simulink model "Lab3Kinematics"  (R2024a)
settings: Solver=VariableStepAuto  StartTime=0.0  StopTime=10.0  RelTol=1e-3
model workspace (MAT data in the model file):
  L = Simulink.Parameter
  L.Value = 0.1
  L.Complexity = 'real'
  L.Dimensions = [1 1]
  L.DataType = 'auto'
  r = Simulink.Parameter
  r.Value = 0.03
  r.Complexity = 'real'
  r.Dimensions = [1 1]
  r.DataType = 'auto'
settings Model: Creator=qjaus  LastModifiedBy=Beast

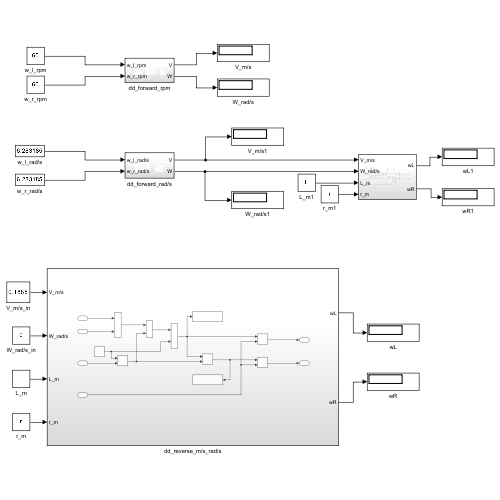
[thumbnail: Simulink's stored preview of the top-level diagram]
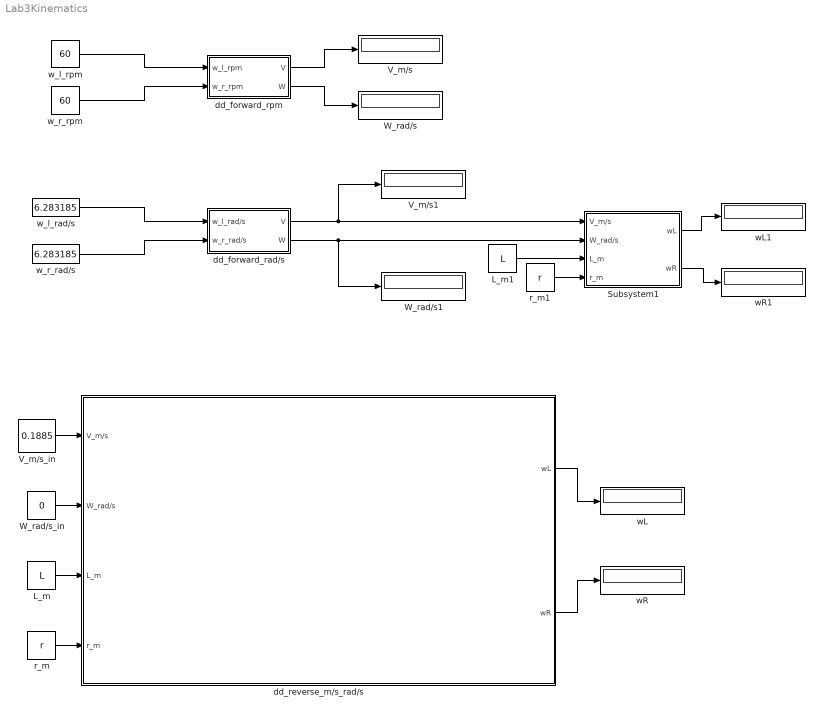
== system Lab3Kinematics ==
  L_m : Constant  Value=L
  L_m1 : Constant  Value=L
  Subsystem1 : Subsystem
  V_m/s : Display
  V_m/s1 : Display
  V_m/s_in : Constant  Value=0.1885
  W_rad/s : Display
  W_rad/s1 : Display
  W_rad/s_in : Constant  Value=0
  dd_forward_rad/s : Subsystem
  dd_forward_rpm : Subsystem
  dd_reverse_m/s_rad/s : Subsystem
  r_m : Constant  Value=r
  r_m1 : Constant  Value=r
  wL : Display
  wL1 : Display
  wR : Display
  wR1 : Display
  w_l_rad/s : Constant  Value=6.283185
  w_l_rpm : Constant  Value=60
  w_r_rad/s : Constant  Value=6.283185
  w_r_rpm : Constant  Value=60
  wires:
  w_l_rpm/1 -> dd_forward_rpm/1(w_l_rpm)
  w_r_rpm/1 -> dd_forward_rpm/2(w_r_rpm)
  dd_forward_rpm/1(V) -> V_m/s/1
  dd_forward_rpm/2(W) -> W_rad/s/1
  dd_forward_rad/s/2(W) -> W_rad/s1/1, Subsystem1/2(W_rad/s)
  w_r_rad/s/1 -> dd_forward_rad/s/2(w_r_rad/s)
  w_l_rad/s/1 -> dd_forward_rad/s/1(w_l_rad/s)
  W_rad/s_in/1 -> dd_reverse_m/s_rad/s/2(W_rad/s)
  L_m/1 -> dd_reverse_m/s_rad/s/3(L_m)
  r_m/1 -> dd_reverse_m/s_rad/s/4(r_m)
  dd_reverse_m/s_rad/s/1(wL) -> wL/1
  dd_reverse_m/s_rad/s/2(wR) -> wR/1
  r_m1/1 -> Subsystem1/4(r_m)
  L_m1/1 -> Subsystem1/3(L_m)
  Subsystem1/1(wL) -> wL1/1
  Subsystem1/2(wR) -> wR1/1
  V_m/s_in/1 -> dd_reverse_m/s_rad/s/1(V_m/s)
  dd_forward_rad/s/1(V) -> V_m/s1/1, Subsystem1/1(V_m/s)

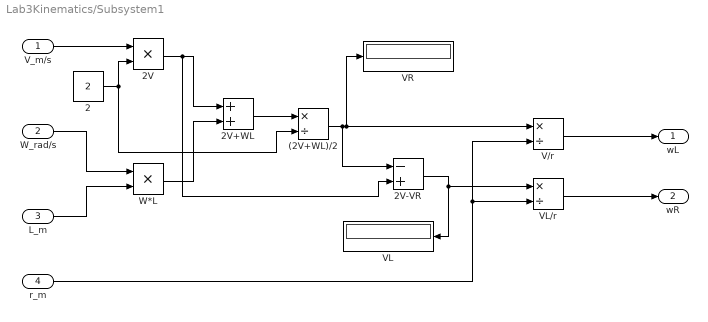
== system Lab3Kinematics/Subsystem1 ==
  V_m/s : Inport
  W_rad/s : Inport  Port=2
  L_m : Inport  Port=3
  r_m : Inport  Port=4
  (2V+WL)/2 : Product  Inputs=*/
  2 : Constant  Value=2
  2V : Product
  2V+WL : Sum
  2V-VR : Sum  Inputs=-+
  V/r : Product  Inputs=*/
  VL : Display
  VL/r : Product  Inputs=*/
  VR : Display
  W*L : Product
  wL : Outport
  wR : Outport  Port=2
  wires:
  2/1 -> 2V/2, (2V+WL)/2/2
  W*L/1 -> 2V+WL/2
  (2V+WL)/2/1 -> 2V-VR/1, VR/1, V/r/1
  r_m/1 -> V/r/2, VL/r/2
  2V-VR/1 -> VL/1, VL/r/1
  2V/1 -> 2V+WL/1, 2V-VR/2
  VL/r/1 -> wR/1
  2V+WL/1 -> (2V+WL)/2/1
  V/r/1 -> wL/1
  V_m/s/1 -> 2V/1
  W_rad/s/1 -> W*L/1
  L_m/1 -> W*L/2

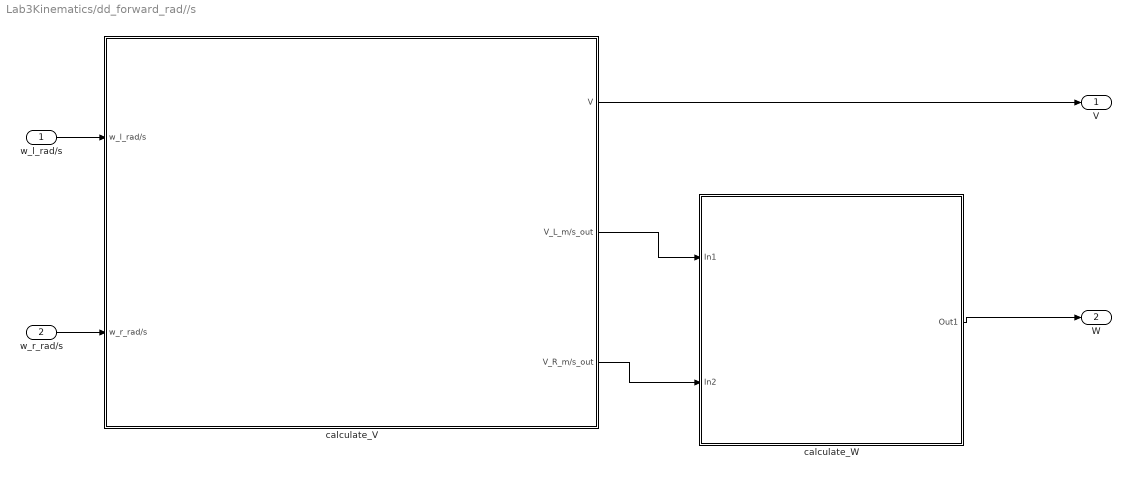
== system Lab3Kinematics/dd_forward_rad//s ==
  w_l_rad/s : Inport
  w_r_rad/s : Inport  Port=2
  calculate_V : Subsystem
  calculate_W : Subsystem
  V : Outport
  W : Outport  Port=2
  wires:
  calculate_V/1(V) -> V/1
  w_r_rad/s/1 -> calculate_V/2(w_r_rad/s)
  w_l_rad/s/1 -> calculate_V/1(w_l_rad/s)
  calculate_V/2(V_L_m/s_out) -> calculate_W/1(In1)
  calculate_W/1(Out1) -> W/1
  calculate_V/3(V_R_m/s_out) -> calculate_W/2(In2)

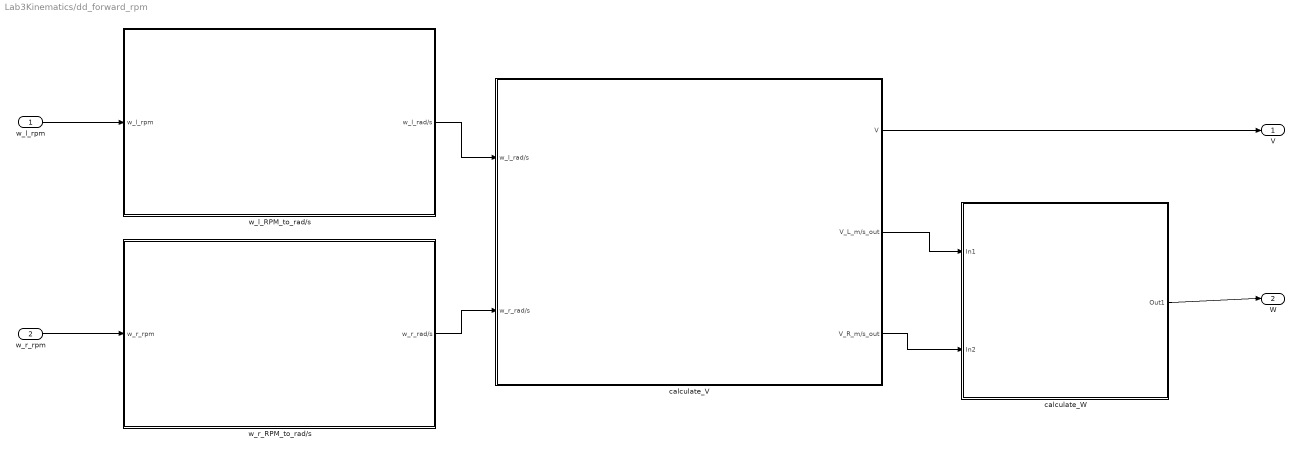
== system Lab3Kinematics/dd_forward_rpm ==
  w_l_rpm : Inport
  w_r_rpm : Inport  Port=2
  calculate_V : Subsystem
  calculate_W : Subsystem
  w_l_RPM_to_rad/s : Subsystem
  w_r_RPM_to_rad/s : Subsystem
  V : Outport
  W : Outport  Port=2
  wires:
  calculate_V/1(V) -> V/1
  w_r_RPM_to_rad/s/1(w_r_rad/s) -> calculate_V/2(w_r_rad/s)
  w_l_RPM_to_rad/s/1(w_l_rad/s) -> calculate_V/1(w_l_rad/s)
  calculate_V/2(V_L_m/s_out) -> calculate_W/1(In1)
  calculate_W/1(Out1) -> W/1
  calculate_V/3(V_R_m/s_out) -> calculate_W/2(In2)
  w_l_rpm/1 -> w_l_RPM_to_rad/s/1(w_l_rpm)
  w_r_rpm/1 -> w_r_RPM_to_rad/s/1(w_r_rpm)

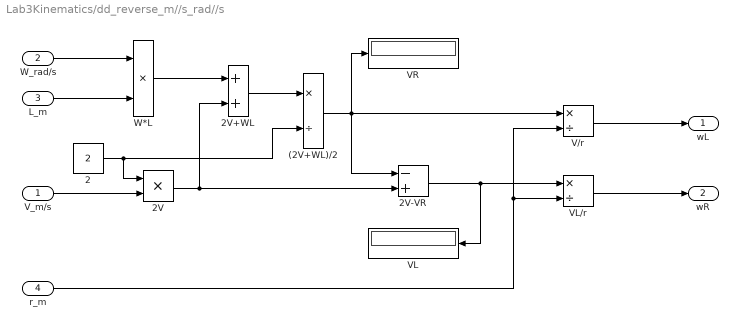
== system Lab3Kinematics/dd_reverse_m//s_rad//s ==
  V_m/s : Inport
  W_rad/s : Inport  Port=2
  L_m : Inport  Port=3
  r_m : Inport  Port=4
  (2V+WL)/2 : Product  Inputs=*/
  2 : Constant  Value=2
  2V : Product
  2V+WL : Sum
  2V-VR : Sum  Inputs=-+
  V/r : Product  Inputs=*/
  VL : Display
  VL/r : Product  Inputs=*/
  VR : Display
  W*L : Product
  wL : Outport
  wR : Outport  Port=2
  wires:
  2/1 -> 2V/1, (2V+WL)/2/2
  W*L/1 -> 2V+WL/1
  (2V+WL)/2/1 -> 2V-VR/1, V/r/1, VR/1
  r_m/1 -> V/r/2, VL/r/2
  2V-VR/1 -> VL/r/1, VL/1
  2V/1 -> 2V+WL/2, 2V-VR/2
  VL/r/1 -> wR/1
  2V+WL/1 -> (2V+WL)/2/1
  V/r/1 -> wL/1
  V_m/s/1 -> 2V/2
  W_rad/s/1 -> W*L/1
  L_m/1 -> W*L/2

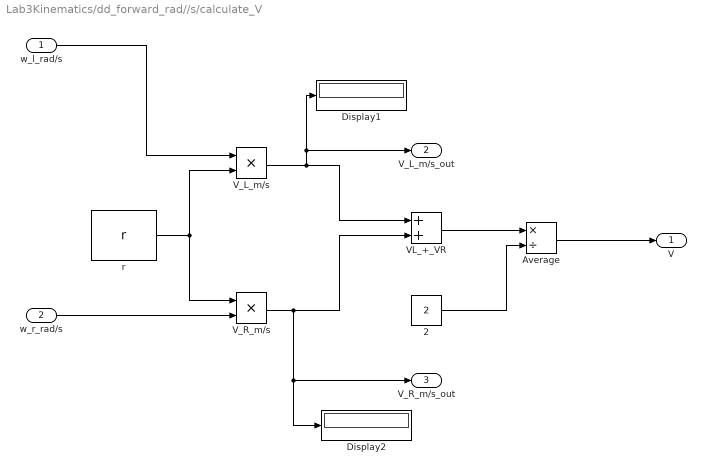
== system Lab3Kinematics/dd_forward_rad//s/calculate_V ==
  w_l_rad/s : Inport
  w_r_rad/s : Inport  Port=2
  2 : Constant  Value=2
  Average : Product  Inputs=*/
  Display1 : Display
  Display2 : Display
  VL_+_VR : Sum
  V_L_m/s : Product
  V_R_m/s : Product
  r : Constant  Value=r
  V : Outport
  V_L_m/s_out : Outport  Port=2
  V_R_m/s_out : Outport  Port=3
  wires:
  w_r_rad/s/1 -> V_R_m/s/2
  VL_+_VR/1 -> Average/1
  r/1 -> V_L_m/s/2, V_R_m/s/1
  V_L_m/s/1 -> Display1/1, V_L_m/s_out/1, VL_+_VR/1
  V_R_m/s/1 -> V_R_m/s_out/1, Display2/1, VL_+_VR/2
  2/1 -> Average/2
  w_l_rad/s/1 -> V_L_m/s/1
  Average/1 -> V/1

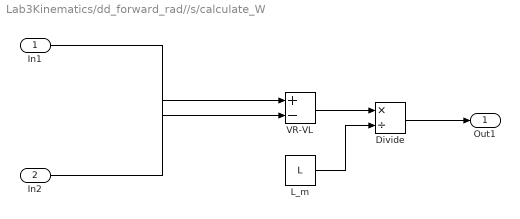
== system Lab3Kinematics/dd_forward_rad//s/calculate_W ==
  In1 : Inport
  In2 : Inport  Port=2
  Divide : Product  Inputs=*/
  L_m : Constant  Value=L
  VR-VL : Sum  Inputs=+-
  Out1 : Outport
  wires:
  L_m/1 -> Divide/2
  VR-VL/1 -> Divide/1
  In2/1 -> VR-VL/1
  In1/1 -> VR-VL/2
  Divide/1 -> Out1/1

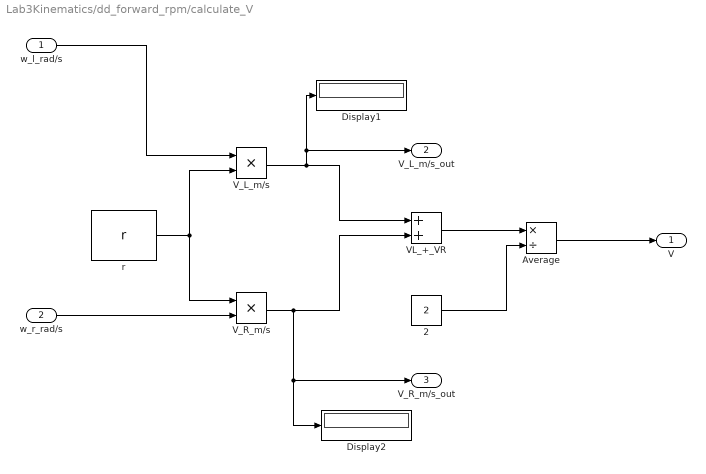
== system Lab3Kinematics/dd_forward_rpm/calculate_V ==
  w_l_rad/s : Inport
  w_r_rad/s : Inport  Port=2
  2 : Constant  Value=2
  Average : Product  Inputs=*/
  Display1 : Display
  Display2 : Display
  VL_+_VR : Sum
  V_L_m/s : Product
  V_R_m/s : Product
  r : Constant  Value=r
  V : Outport
  V_L_m/s_out : Outport  Port=2
  V_R_m/s_out : Outport  Port=3
  wires:
  w_r_rad/s/1 -> V_R_m/s/2
  VL_+_VR/1 -> Average/1
  r/1 -> V_L_m/s/2, V_R_m/s/1
  V_L_m/s/1 -> Display1/1, V_L_m/s_out/1, VL_+_VR/1
  V_R_m/s/1 -> V_R_m/s_out/1, Display2/1, VL_+_VR/2
  2/1 -> Average/2
  w_l_rad/s/1 -> V_L_m/s/1
  Average/1 -> V/1

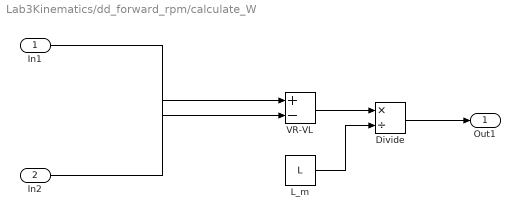
== system Lab3Kinematics/dd_forward_rpm/calculate_W ==
  In1 : Inport
  In2 : Inport  Port=2
  Divide : Product  Inputs=*/
  L_m : Constant  Value=L
  VR-VL : Sum  Inputs=+-
  Out1 : Outport
  wires:
  L_m/1 -> Divide/2
  VR-VL/1 -> Divide/1
  In2/1 -> VR-VL/1
  In1/1 -> VR-VL/2
  Divide/1 -> Out1/1

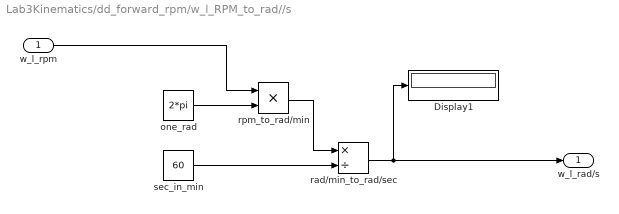
== system Lab3Kinematics/dd_forward_rpm/w_l_RPM_to_rad//s ==
  w_l_rpm : Inport
  Display1 : Display
  one_rad : Constant  Value=2*pi
  rad/min_to_rad/sec : Product  Inputs=*/
  rpm_to_rad/min : Product
  sec_in_min : Constant  Value=60
  w_l_rad/s : Outport
  wires:
  one_rad/1 -> rpm_to_rad/min/2
  rad/min_to_rad/sec/1 -> w_l_rad/s/1, Display1/1
  sec_in_min/1 -> rad/min_to_rad/sec/2
  rpm_to_rad/min/1 -> rad/min_to_rad/sec/1
  w_l_rpm/1 -> rpm_to_rad/min/1

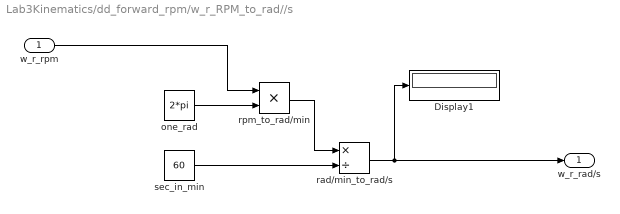
== system Lab3Kinematics/dd_forward_rpm/w_r_RPM_to_rad//s ==
  w_r_rpm : Inport
  Display1 : Display
  one_rad : Constant  Value=2*pi
  rad/min_to_rad/s : Product  Inputs=*/
  rpm_to_rad/min : Product
  sec_in_min : Constant  Value=60
  w_r_rad/s : Outport
  wires:
  one_rad/1 -> rpm_to_rad/min/2
  rad/min_to_rad/s/1 -> w_r_rad/s/1, Display1/1
  sec_in_min/1 -> rad/min_to_rad/s/2
  rpm_to_rad/min/1 -> rad/min_to_rad/s/1
  w_r_rpm/1 -> rpm_to_rad/min/1
